simulink model "rx2"  (R2022b)
settings: Solver=FixedStepDiscrete  StartTime=0.0  StopTime=3.3E6  FixedStep=1  RelTol=1e-3  EnableMultiTasking=on
model workspace (MAT data in the model file):
  mwTaskManagerKernelLatency = 0
undefined symbols (not defined in the file or in its folder): Add, jsin, magnitude, rom_pilot_conj_tt, Shift
libraries: hdlsllib x3231, whdlutilities x525, simulink x260, whdlmod x112, whdledac x26, dsphdlmathfun2 x24, commchan3 x1
(part 16 of 59)

== system rx2/process9/decoder/p-p ==
  data_in : Inport  OutDataTypeStr=boolean  PortDimensions=64
  start_in : Inport  Port=2  OutDataTypeStr=boolean  PortDimensions=1
  valid : Inport  Port=3  OutDataTypeStr=boolean  PortDimensions=1
  Compare To Constant : hdlsllib/Logic and Bit Operations/Compare To Constant  relop===  const=64  OutDataTypeStr=boolean
  Compare To Constant1 : hdlsllib/Logic and Bit Operations/Compare To Constant  relop=<=  const=72  OutDataTypeStr=boolean
  Compare To Constant2 : hdlsllib/Logic and Bit Operations/Compare To Constant  relop===  const=1  OutDataTypeStr=boolean
  Compare To Constant3 : hdlsllib/Logic and Bit Operations/Compare To Constant  relop===  const=528  OutDataTypeStr=boolean
  Compare To Constant4 : hdlsllib/Logic and Bit Operations/Compare To Constant  relop=<=  const=528  OutDataTypeStr=boolean
  Delay : Delay  DelayLength=1  InitialCondition=0
  Delay1 : Delay  DelayLength=1  InitialCondition=0
  Ground : Ground
  HDL Counter : hdlsllib/Sources/HDL Counter  CountType=Count limited  CountInit=0  CountStep=1  CountMax=2000  CountFromType=Specify  CountFrom=0  CountResetPort=on  CountLoadPort=off  CountEnbPort=on  CountDirPort=off  CountHitOutputPort=off  CountDataType=Unsigned  CountWordLen=16  CountFracLen=0  CountSampTime=1
  HDL Counter1 : hdlsllib/Sources/HDL Counter  CountType=Count limited  CountInit=1  CountStep=1  CountMax=64  CountFromType=Specify  CountFrom=1  CountResetPort=on  CountLoadPort=off  CountEnbPort=on  CountDirPort=off  CountHitOutputPort=off  CountDataType=Unsigned  CountWordLen=16  CountFracLen=0  CountSampTime=1
  HDL Counter2 : hdlsllib/Sources/HDL Counter  CountType=Count limited  CountInit=0  CountStep=1  CountMax=100  CountFromType=Specify  CountFrom=0  CountResetPort=on  CountLoadPort=off  CountEnbPort=on  CountDirPort=off  CountHitOutputPort=off  CountDataType=Unsigned  CountWordLen=16  CountFracLen=0  CountSampTime=1
  HDL Counter3 : hdlsllib/Sources/HDL Counter  CountType=Count limited  CountInit=1  CountStep=1  CountMax=64*2  CountFromType=Initial value  CountFrom=1  CountResetPort=on  CountLoadPort=off  CountEnbPort=on  CountDirPort=off  CountHitOutputPort=off  CountDataType=Unsigned  CountWordLen=8  CountFracLen=0  CountSampTime=1
  HDL Counter4 : hdlsllib/Sources/HDL Counter  CountType=Count limited  CountInit=0  CountStep=1  CountMax=1000  CountFromType=Initial value  CountFrom=0  CountResetPort=on  CountLoadPort=off  CountEnbPort=on  CountDirPort=off  CountHitOutputPort=off  CountDataType=Unsigned  CountWordLen=16  CountFracLen=0  CountSampTime=1
  HDL Counter5 : hdlsllib/Sources/HDL Counter  CountType=Count limited  CountInit=1  CountStep=1  CountMax=1000  CountFromType=Initial value  CountFrom=1  CountResetPort=on  CountLoadPort=off  CountEnbPort=on  CountDirPort=off  CountHitOutputPort=off  CountDataType=Unsigned  CountWordLen=16  CountFracLen=0  CountSampTime=1
  Logical Operator1 : Logic  Operator=NOT  AllPortsSameDT=off  OutDataTypeStr=boolean
  Logical Operator2 : Logic  Operator=NOT  AllPortsSameDT=off  OutDataTypeStr=boolean
  Logical Operator3 : Logic  AllPortsSameDT=off  OutDataTypeStr=boolean
  Logical Operator5 : Logic  Operator=NOT  AllPortsSameDT=off  OutDataTypeStr=boolean
  Logical Operator6 : Logic  AllPortsSameDT=off  OutDataTypeStr=boolean
  Sample Control Bus Creator : whdlutilities/Sample Control Bus Creator
  Subsystem : Subsystem  mask{valid_length=20*64}
      mask prompts: valid_length "The length of valid"
      mask DialogControl Control2 Prompt: Latency=2
  Subsystem2 : Subsystem  mask{data_type=boolean, address_len=16}
      mask prompts: data_type "the type of input data"; address_len "the length of address"
      mask DialogControl ParameterGroupVar Prompt: 参数
  Switch : Switch  Criteria=u2 ~= 0  SaturateOnIntegerOverflow=off  InputSameDT=off
  p_s_new : Subsystem
  data : Outport
  ctrl : Outport  Port=2
  wires:
  Ground/1 -> Switch/3
  Switch/1 -> data/1
  Subsystem/3(end_out) -> p_s_new/3(end)
  p_s_new/1(data_out) -> Delay1/1
  Subsystem2/1(rd_dout) -> p_s_new/1(data_in)
  Subsystem/1(valid_out) -> HDL Counter1/2, Logical Operator1/1, HDL Counter3/2, Logical Operator2/1, Logical Operator3/1, p_s_new/2(valid)
  Logical Operator6/1 -> HDL Counter4/2, Delay/1
  Compare To Constant4/1 -> Logical Operator6/1
  HDL Counter5/1 -> Compare To Constant4/1
  Sample Control Bus Creator/1 -> ctrl/1
  Delay1/1 -> Switch/1
  Delay/1 -> Sample Control Bus Creator/3, Switch/2
  Compare To Constant3/1 -> HDL Counter4/1, Sample Control Bus Creator/2
  Compare To Constant2/1 -> Sample Control Bus Creator/1
  HDL Counter1/1 -> Compare To Constant/1
  Compare To Constant1/1 -> Logical Operator3/2
  HDL Counter3/1 -> Compare To Constant1/1
  HDL Counter2/1 -> Subsystem2/4(rd_addr)
  data_in/1 -> Subsystem2/1(data1)
  Logical Operator5/1 -> HDL Counter/1
  Logical Operator2/1 -> HDL Counter3/1, HDL Counter5/1
  Compare To Constant/1 -> HDL Counter2/2
  start_in/1 -> Subsystem/1(start)
  HDL Counter/1 -> Subsystem2/2(wr_addr)
  valid/1 -> Logical Operator5/1, Subsystem2/3(wr_en1), HDL Counter/2
  Logical Operator3/1 -> Logical Operator6/2, HDL Counter5/2
  Logical Operator1/1 -> HDL Counter1/1, HDL Counter2/1
  HDL Counter4/1 -> Compare To Constant2/1, Compare To Constant3/1

== system rx2/process9/decoder/rate recover ==
  demod : Inport
  valid_in : Inport  Port=2
  start_in : Inport  Port=3
  Compare To Constant : hdlsllib/Logic and Bit Operations/Compare To Constant  relop=<=  const=384  OutDataTypeStr=boolean
  Compare To Constant1 : hdlsllib/Logic and Bit Operations/Compare To Constant  relop=>=  const=577  OutDataTypeStr=boolean
  Compare To Constant2 : hdlsllib/Logic and Bit Operations/Compare To Constant  relop=<=  const=1776  OutDataTypeStr=boolean
  Compare To Constant3 : hdlsllib/Logic and Bit Operations/Compare To Constant  relop=>=  const=385  OutDataTypeStr=boolean
  Compare To Constant4 : hdlsllib/Logic and Bit Operations/Compare To Constant  relop=<=  const=576  OutDataTypeStr=boolean
  Compare To Constant5 : hdlsllib/Logic and Bit Operations/Compare To Constant  relop=>=  const=1777  OutDataTypeStr=boolean
  Compare To Constant6 : hdlsllib/Logic and Bit Operations/Compare To Constant  relop=<=  const=3600  OutDataTypeStr=boolean
  Constant : Constant  Value=0
  Constant1 : Constant  Value=0
  Delay{,1..4} (5 alike) : Delay  InitialCondition=0
  HDL Counter : hdlsllib/Sources/HDL Counter  CountType=Count limited  CountInit=1  CountStep=1  CountMax=10000  CountFromType=Initial value  CountFrom=1  CountResetPort=on  CountLoadPort=off  CountEnbPort=on  CountDirPort=off  CountHitOutputPort=off  CountDataType=Unsigned  CountWordLen=16  CountFracLen=0  CountSampTime=1
  HDL Counter1 : hdlsllib/Sources/HDL Counter  CountType=Count limited  CountInit=0  CountStep=1  CountMax=10000  CountFromType=Initial value  CountFrom=0  CountResetPort=on  CountLoadPort=off  CountEnbPort=on  CountDirPort=off  CountHitOutputPort=off  CountDataType=Unsigned  CountWordLen=16  CountFracLen=0  CountSampTime=1
  HDL Counter3 : hdlsllib/Sources/HDL Counter  CountType=Count limited  CountInit=1  CountStep=1  CountMax=10000  CountFromType=Initial value  CountFrom=1  CountResetPort=on  CountLoadPort=off  CountEnbPort=on  CountDirPort=off  CountHitOutputPort=off  CountDataType=Unsigned  CountWordLen=16  CountFracLen=0  CountSampTime=1
  Logical Operator : Logic  Operator=NOT  AllPortsSameDT=off  OutDataTypeStr=boolean
  Logical Operator{1,3..4,6..7} (5 alike) : Logic  AllPortsSameDT=off  OutDataTypeStr=boolean
  Logical Operator5 : Logic  Operator=OR  AllPortsSameDT=off  OutDataTypeStr=boolean
  Logical Operator8 : Logic  Operator=NOT  AllPortsSameDT=off  OutDataTypeStr=boolean
  Simple Dual Port RAM : hdlsllib/HDL RAMs/Simple Dual Port RAM  ram_size=16
  Subsystem : Subsystem  mask{valid_length=3600}
      mask prompts: valid_length "The length of valid"
      mask DialogControl Control2 Prompt: Latency=2
  Switch : Switch  Criteria=u2 ~= 0  SaturateOnIntegerOverflow=off  InputSameDT=off
  Switch1 : Switch  Criteria=u2 ~= 0  OutDataTypeStr=fixdt(1,16,9)  SaturateOnIntegerOverflow=off  InputSameDT=off
  rate_recover : Outport  PortDimensions=1
  start_out : Outport  Port=2  OutDataTypeStr=boolean
  end_out : Outport  Port=3  OutDataTypeStr=boolean
  valid_out : Outport  Port=4  OutDataTypeStr=boolean
  wires:
  Compare To Constant5/1 -> Logical Operator4/1
  Logical Operator3/1 -> Delay3/1
  Subsystem/1(valid_out) -> Logical Operator8/1, Logical Operator6/2, Delay/1, HDL Counter3/2
  Constant1/1 -> Switch1/1
  Subsystem/2(start_out) -> Delay1/1  "start"
  Logical Operator/1 -> HDL Counter/1
  Logical Operator1/1 -> Logical Operator5/2
  Compare To Constant3/1 -> Logical Operator3/1
  Subsystem/3(end_out) -> Delay2/1  "end"
  HDL Counter/1 -> Simple Dual Port RAM/2  "wr_addr"
  Compare To Constant6/1 -> Logical Operator4/2
  Compare To Constant1/1 -> Logical Operator1/1
  Compare To Constant2/1 -> Logical Operator1/2
  valid_in/1 -> Simple Dual Port RAM/3, HDL Counter/2, Logical Operator/1
  Delay1/1 -> start_out/1  "start_out"
  Logical Operator7/1 -> Delay4/1  "3"
  Simple Dual Port RAM/1 -> Switch/3  "rd_dout"
  start_in/1 -> Subsystem/1(start)
  Compare To Constant4/1 -> Logical Operator3/2
  Logical Operator4/1 -> Logical Operator7/1
  Constant/1 -> Switch/1
  Switch/1 -> Switch1/3  "2_out"
  Switch1/1 -> rate_recover/1  "data_out"
  Logical Operator5/1 -> Logical Operator6/1
  Compare To Constant/1 -> Logical Operator5/1
  Delay2/1 -> end_out/1  "end_out"
  demod/1 -> Simple Dual Port RAM/1
  Delay/1 -> Logical Operator7/2, valid_out/1  "valid_out"
  Logical Operator8/1 -> HDL Counter1/1, HDL Counter3/1
  HDL Counter3/1 -> Compare To Constant1/1, Compare To Constant/1, Compare To Constant6/1, Compare To Constant5/1, Compare To Constant4/1, Compare To Constant3/1, Compare To Constant2/1  "count"
  Delay3/1 -> Switch/2  "2"
  Delay4/1 -> Switch1/2  "3"
  Logical Operator6/1 -> HDL Counter1/2  "1"
  HDL Counter1/1 -> Simple Dual Port RAM/4  "rd_addr"

== system rx2/process9/decoder/s-p ==
  data_in : Inport
  valid_in : Inport  Port=2
  Compare To Constant1 : hdlsllib/Logic and Bit Operations/Compare To Constant  relop=<=  const=64  OutDataTypeStr=boolean
  Compare To Constant2 : hdlsllib/Logic and Bit Operations/Compare To Constant  relop===  const=2  OutDataTypeStr=boolean
  Compare To Constant3 : hdlsllib/Logic and Bit Operations/Compare To Constant  relop===  const=3  OutDataTypeStr=boolean
  Compare To Constant4 : hdlsllib/Logic and Bit Operations/Compare To Constant  relop===  const=1  OutDataTypeStr=boolean
  Compare To Constant5 : hdlsllib/Logic and Bit Operations/Compare To Constant  relop===  const=100  OutDataTypeStr=boolean
  Constant2 : Constant  Value=2  OutDataTypeStr=uint8
  Constant3 : Constant  Value=zeros(1,56)  OutDataTypeStr=fixdt(1,16,9)
  Delay1 : Delay  DelayLength=1  InitialCondition=0
  Delay4 : Delay  DelayLength=1  InitialCondition=0
  HDL Counter : hdlsllib/Sources/HDL Counter  CountType=Count limited  CountInit=1  CountStep=1  CountMax=72  CountFromType=Initial value  CountFrom=1  CountResetPort=on  CountLoadPort=off  CountEnbPort=on  CountDirPort=off  CountHitOutputPort=off  CountDataType=Unsigned  CountWordLen=8  CountFracLen=0  CountSampTime=1
  HDL Counter1 : hdlsllib/Sources/HDL Counter  CountType=Count limited  CountInit=1  CountStep=1  CountMax=72  CountFromType=Initial value  CountFrom=1  CountResetPort=on  CountLoadPort=off  CountEnbPort=on  CountDirPort=off  CountHitOutputPort=off  CountDataType=Unsigned  CountWordLen=8  CountFracLen=0  CountSampTime=1
  HDL Counter2 : hdlsllib/Sources/HDL Counter  CountType=Count limited  CountInit=1  CountStep=1  CountMax=72  CountFromType=Initial value  CountFrom=1  CountResetPort=on  CountLoadPort=off  CountEnbPort=on  CountDirPort=off  CountHitOutputPort=off  CountDataType=Unsigned  CountWordLen=8  CountFracLen=0  CountSampTime=1
  HDL Counter3 : hdlsllib/Sources/HDL Counter  CountType=Count limited  CountInit=0  CountStep=1  CountMax=200  CountFromType=Initial value  CountFrom=0  CountResetPort=on  CountLoadPort=off  CountEnbPort=on  CountDirPort=off  CountHitOutputPort=off  CountDataType=Unsigned  CountWordLen=8  CountFracLen=0  CountSampTime=1
  Logical Operator{1,5..6,8} (4 alike) : Logic  Operator=NOT  AllPortsSameDT=off  OutDataTypeStr=boolean
  Logical Operator2 : Logic  Operator=XOR  AllPortsSameDT=off  OutDataTypeStr=boolean
  Logical Operator3 : Logic  AllPortsSameDT=off  OutDataTypeStr=boolean
  Logical Operator4 : Logic  AllPortsSameDT=off  OutDataTypeStr=boolean
  Mod : Math  Operator=mod
  Mux : Mux  Inputs=2
  S-P : Subsystem  mask{data_len=64}
      mask prompts: data_len "the length of parallel"
      mask DialogControl ParameterGroupVar Prompt: 参数
  S-P2 : Subsystem  mask{data_len=8}
      mask prompts: data_len "the length of parallel"
      mask DialogControl ParameterGroupVar Prompt: 参数
  Sample Control Bus Creator : whdlutilities/Sample Control Bus Creator
  Switch1 : Switch  Criteria=u2 ~= 0  OutDataTypeStr=Inherit: Inherit via back propagation  SaturateOnIntegerOverflow=off  InputSameDT=off
  data_out : Outport
  ctrl_out : Outport  Port=2
  wires:
  Compare To Constant1/1 -> Logical Operator8/1, Logical Operator3/2
  Logical Operator2/1 -> Delay1/1, HDL Counter3/2  "valid"
  Logical Operator4/1 -> Sample Control Bus Creator/1  "start"
  HDL Counter/1 -> Compare To Constant1/1
  Compare To Constant2/1 -> Logical Operator2/1, Delay4/1
  S-P2/2(valid_out) -> HDL Counter2/2, Logical Operator6/1
  HDL Counter1/1 -> Compare To Constant2/1
  data_in/1 -> S-P2/1(data_in), S-P/1(data_in)
  valid_in/1 -> Logical Operator1/1, Logical Operator3/1, HDL Counter/2
  Sample Control Bus Creator/1 -> ctrl_out/1
  Constant3/1 -> Mux/2
  HDL Counter3/1 -> Mod/1, Compare To Constant4/1, Compare To Constant5/1
  Compare To Constant3/1 -> Logical Operator2/2
  Mod/1 -> Switch1/2
  Switch1/1 -> data_out/1
  Constant2/1 -> Mod/2
  S-P2/1(data_out) -> Mux/1
  Mux/1 -> Switch1/3
  HDL Counter2/1 -> Compare To Constant3/1
  Logical Operator8/1 -> S-P2/2(valid_in)
  S-P/2(valid_out) -> HDL Counter1/2, Logical Operator5/1  "validout"
  S-P/1(data_out) -> Switch1/1
  Logical Operator3/1 -> S-P/2(valid_in)
  Logical Operator1/1 -> HDL Counter/1
  Logical Operator5/1 -> HDL Counter1/1
  Logical Operator6/1 -> HDL Counter2/1
  Compare To Constant5/1 -> Sample Control Bus Creator/2, HDL Counter3/1  "start"
  Compare To Constant4/1 -> Logical Operator4/2
  Delay4/1 -> Logical Operator4/1
  Delay1/1 -> Sample Control Bus Creator/3

== system rx2/process9/decoder/soft demodule ==
  nVar_tt : Inport  OutDataTypeStr=fixdt(0,16,12)
  G_k_1 : Inport  Port=2
  r_k : Inport  Port=3
  start : Inport  Port=4
  valid : Inport  Port=5
  Complex to Real-Imag : ComplexToRealImag
  Constant1 : Constant  Value=2  OutDataTypeStr=uint16
  Constant2 : Constant  Value=2  OutDataTypeStr=uint16
  Constant3 : Constant  Value=0  OutDataTypeStr=uint16
  Constant4 : Constant  Value=0  OutDataTypeStr=uint16
  Data Type Conversion2 : DataTypeConversion  OutDataTypeStr=boolean  SaturateOnIntegerOverflow=off  RndMeth=Floor
  Delay1 : Delay  InitialCondition=0
  Delay2 : Delay  DelayLength=1  InitialCondition=0
  Delay3 : Delay  InitialCondition=0
  Delay4 : Delay  InitialCondition=0
  HDL Counter : hdlsllib/Sources/HDL Counter  CountType=Count limited  CountInit=1  CountStep=1  CountMax=2000  CountFromType=Initial value  CountFrom=1  CountResetPort=on  CountLoadPort=off  CountEnbPort=on  CountDirPort=off  CountHitOutputPort=off  CountDataType=Unsigned  CountWordLen=16  CountFracLen=0  CountSampTime=1
  HDL Counter2 : hdlsllib/Sources/HDL Counter  CountType=Count limited  CountInit=1  CountStep=1  CountMax=2000  CountFromType=Initial value  CountFrom=1  CountResetPort=on  CountLoadPort=off  CountEnbPort=on  CountDirPort=off  CountHitOutputPort=off  CountDataType=Unsigned  CountWordLen=16  CountFracLen=0  CountSampTime=1
  HDL Counter3 : hdlsllib/Sources/HDL Counter  CountType=Count limited  CountInit=0  CountStep=1  CountMax=2000  CountFromType=Initial value  CountFrom=0  CountResetPort=on  CountLoadPort=off  CountEnbPort=on  CountDirPort=off  CountHitOutputPort=off  CountDataType=Unsigned  CountWordLen=16  CountFracLen=0  CountSampTime=1
  HDL Counter5 : hdlsllib/Sources/HDL Counter  CountType=Count limited  CountInit=0  CountStep=1  CountMax=2000  CountFromType=Initial value  CountFrom=0  CountResetPort=on  CountLoadPort=off  CountEnbPort=on  CountDirPort=off  CountHitOutputPort=off  CountDataType=Unsigned  CountWordLen=16  CountFracLen=0  CountSampTime=1
  Logical Operator2 : Logic  AllPortsSameDT=off  OutDataTypeStr=boolean
  Logical Operator3 : Logic  Operator=NOT  AllPortsSameDT=off  OutDataTypeStr=boolean
  Logical Operator4 : Logic  Operator=NOT  AllPortsSameDT=off  OutDataTypeStr=boolean
  Logical Operator5 : Logic  Operator=NOT  AllPortsSameDT=off  OutDataTypeStr=boolean
  Logical Operator6 : Logic  Operator=XOR  AllPortsSameDT=off  OutDataTypeStr=boolean
  Math Reciprocal2 : Math  Operator=reciprocal  SignedPower=on  OutDataTypeStr=fixdt(1,16,12)
  Mod : Math  Operator=mod  SignedPower=on
  Product : Product
  Product1 : Product
  Product10 : Product  OutDataTypeStr=fixdt(1,35,24)
  Product2 : Product  OutDataTypeStr=fixdt(1,35,24)
  Simple Dual Port RAM : hdlsllib/HDL RAMs/Simple Dual Port RAM  ram_size=16
  Simple Dual Port RAM1 : hdlsllib/HDL RAMs/Simple Dual Port RAM  ram_size=16
  Subsystem : Subsystem  mask{valid_length=demod_length}
      mask prompts: valid_length "The length of valid"
      mask DialogControl Control2 Prompt: Latency=2
  Switch : Switch  Criteria=u2 ~= 0  SaturateOnIntegerOverflow=off  InputSameDT=off
  Switch1 : Switch  Criteria=u2 ~= 0  SaturateOnIntegerOverflow=off  InputSameDT=off
  Switch2 : Switch  Criteria=u2 ~= 0  SaturateOnIntegerOverflow=off  InputSameDT=off
  demod : Outport  OutDataTypeStr=fixdt(1,16,9)  VectorParamsAs1DForOutWhenUnconnected=off
  valid_out : Outport  Port=2  OutDataTypeStr=boolean  VectorParamsAs1DForOutWhenUnconnected=off
  start_out : Outport  Port=3  OutDataTypeStr=boolean  VectorParamsAs1DForOutWhenUnconnected=off
  end_out : Outport  Port=4  OutDataTypeStr=boolean  VectorParamsAs1DForOutWhenUnconnected=off
  wires:
  valid/1 -> Switch2/2, Switch1/2, Simple Dual Port RAM1/3, Simple Dual Port RAM/3, HDL Counter2/2, Logical Operator4/1  "valid_tt"
  start/1 -> Subsystem/1(start)
  Logical Operator2/1 -> Logical Operator6/2, HDL Counter3/2  "mod_1"
  Complex to Real-Imag/2 -> Product1/2  "r_k_imag"
  Subsystem/1(valid_out) -> Delay1/1, HDL Counter/2, Logical Operator3/1, Logical Operator2/2, Logical Operator6/1, Logical Operator5/1
  Product/1 -> Switch1/1  "demod_1"
  Product1/1 -> Switch2/1  "demod_0"
  Switch/1 -> demod/1  "demod"
  Mod/1 -> Data Type Conversion2/1  "mod"
  Logical Operator6/1 -> Delay2/1, HDL Counter5/2  "mod_0"
  Complex to Real-Imag/1 -> Product/2  "r_k_real"
  Logical Operator4/1 -> HDL Counter2/1
  HDL Counter3/1 -> Simple Dual Port RAM/4  "rd_addr1"
  Logical Operator5/1 -> HDL Counter5/1, HDL Counter3/1  "rst"
  Logical Operator3/1 -> HDL Counter/1
  Constant1/1 -> Mod/2
  HDL Counter5/1 -> Simple Dual Port RAM1/4  "rd_addr0"
  Simple Dual Port RAM/1 -> Switch/1  "demod_11"
  HDL Counter2/1 -> Simple Dual Port RAM1/2, Simple Dual Port RAM/2  "wr_addr"
  Simple Dual Port RAM1/1 -> Switch/3  "demod_00"
  Data Type Conversion2/1 -> Logical Operator2/1
  Delay1/1 -> valid_out/1  "valid_out"
  HDL Counter/1 -> Mod/1  "count"
  nVar_tt/1 -> Math Reciprocal2/1  "nvar"
  G_k_1/1 -> Product10/2  "G_k_1"
  r_k/1 -> Complex to Real-Imag/1  "r_k"
  Subsystem/2(start_out) -> Delay3/1
  Subsystem/3(end_out) -> Delay4/1
  Delay2/1 -> Switch/2
  Delay3/1 -> start_out/1  "start_out"
  Delay4/1 -> end_out/1  "end_out"
  Math Reciprocal2/1 -> Product10/1  "nvar"
  Product10/1 -> Product2/2
  Product2/1 -> Product1/1, Product/1
  Constant2/1 -> Product2/1
  Constant3/1 -> Switch1/3
  Switch1/1 -> Simple Dual Port RAM/1  "demod1"
  Constant4/1 -> Switch2/3
  Switch2/1 -> Simple Dual Port RAM1/1  "demod0"

== system rx2/process9/decoder/synchronization ==
  chan_est_tt : Inport
  rxSig_tt : Inport  Port=2
  port1_ctrl : Inport  Port=3  OutDataTypeStr=Bus: BUSOFDM1
  port2_ctrl : Inport  Port=4  OutDataTypeStr=Bus: BUSOFDM1
  Bus Selector1 : BusSelector  OutputSignals=signal1,signal2,signal3,signal4,signal5,signal6,signal7,signal8
  Bus Selector2 : BusSelector  OutputSignals=OFDM_ctrl_bf1_process1,OFDM_ctrl_bf1_process2,OFDM_ctrl_bf1_process3,OFDM_ctrl_bf1_process4,OFDM_ctrl_bf1_process5,OFDM_ctrl_bf1_process6,OFDM_ctrl_bf1_process7,OFDM_ctrl_bf1_process8
  Demux : Demux  Outputs=8
  Demux1 : Demux  Outputs=8
  Mux : Mux  Inputs=8
  Mux1 : Mux  Inputs=8
  data_synchronization1 : Subsystem
  data_synchronization2 : Subsystem
  data_synchronization3 : Subsystem
  data_synchronization4 : Subsystem
  data_synchronization5 : Subsystem
  data_synchronization6 : Subsystem
  data_synchronization7 : Subsystem
  data_synchronization8 : Subsystem
  port1_syn : Outport
  port2_syn : Outport  Port=2
  valid_syn : Outport  Port=3
  wires:
  Bus Selector2/3 -> data_synchronization8/4(port2_ctrl)  "<OFDM_ctrl_bf1_process3>"
  Bus Selector2/4 -> data_synchronization7/4(port2_ctrl)  "<OFDM_ctrl_bf1_process4>"
  Bus Selector2/5 -> data_synchronization6/4(port2_ctrl)  "<OFDM_ctrl_bf1_process5>"
  Bus Selector2/6 -> data_synchronization5/4(port2_ctrl)  "<OFDM_ctrl_bf1_process6>"
  Bus Selector2/7 -> data_synchronization4/4(port2_ctrl)  "<OFDM_ctrl_bf1_process7>"
  Bus Selector2/8 -> data_synchronization3/4(port2_ctrl)  "<OFDM_ctrl_bf1_process8>"
  Bus Selector2/2 -> data_synchronization2/4(port2_ctrl)  "<OFDM_ctrl_bf1_process2>"
  Bus Selector2/1 -> data_synchronization1/4(port2_ctrl)  "<OFDM_ctrl_bf1_process1>"
  port2_ctrl/1 -> Bus Selector2/1
  Bus Selector1/8 -> data_synchronization8/3(port1_ctrl)  "<signal8>"
  Bus Selector1/7 -> data_synchronization7/3(port1_ctrl)  "<signal7>"
  Bus Selector1/6 -> data_synchronization6/3(port1_ctrl)  "<signal6>"
  Bus Selector1/5 -> data_synchronization5/3(port1_ctrl)  "<signal5>"
  Bus Selector1/4 -> data_synchronization4/3(port1_ctrl)  "<signal4>"
  Bus Selector1/3 -> data_synchronization3/3(port1_ctrl)  "<signal3>"
  Bus Selector1/2 -> data_synchronization2/3(port1_ctrl)  "<signal2>"
  Bus Selector1/1 -> data_synchronization1/3(port1_ctrl)  "<signal1>"
  port1_ctrl/1 -> Bus Selector1/1
  rxSig_tt/1 -> Demux1/1
  data_synchronization6/3(valid_syn) -> ?
  chan_est_tt/1 -> Demux/1
  data_synchronization4/4(start_syn) -> ?
  data_synchronization2/3(valid_syn) -> ?
  data_synchronization4/3(valid_syn) -> ?
  data_synchronization6/4(start_syn) -> ?
  data_synchronization7/3(valid_syn) -> ?
  data_synchronization3/3(valid_syn) -> ?
  data_synchronization5/3(valid_syn) -> ?
  data_synchronization8/4(start_syn) -> ?
  Demux1/5 -> data_synchronization5/2(port2)
  Demux1/3 -> data_synchronization3/2(port2)
  data_synchronization2/4(start_syn) -> ?
  data_synchronization3/2(port2_syn) -> Mux1/3
  data_synchronization7/1(port1_syn) -> Mux/7
  Demux1/1 -> data_synchronization1/2(port2)
  Demux/8 -> data_synchronization8/1(port1)
  data_synchronization1/1(port1_syn) -> Mux/1
  Demux/3 -> data_synchronization3/1(port1)
  data_synchronization3/4(start_syn) -> ?
  data_synchronization1/3(valid_syn) -> valid_syn/1
  data_synchronization1/2(port2_syn) -> Mux1/1
  Demux/4 -> data_synchronization4/1(port1)
  data_synchronization5/4(start_syn) -> ?
  data_synchronization8/1(port1_syn) -> Mux/8
  Demux/6 -> data_synchronization6/1(port1)
  data_synchronization7/2(port2_syn) -> Mux1/7
  data_synchronization6/1(port1_syn) -> Mux/6
  Demux/7 -> data_synchronization7/1(port1)
  Demux/1 -> data_synchronization1/1(port1)
  data_synchronization4/2(port2_syn) -> Mux1/4
  data_synchronization4/1(port1_syn) -> Mux/4
  data_synchronization5/2(port2_syn) -> Mux1/5
  data_synchronization5/1(port1_syn) -> Mux/5
  Mux1/1 -> port2_syn/1
  Demux1/4 -> data_synchronization4/2(port2)
  Demux1/6 -> data_synchronization6/2(port2)
  data_synchronization8/2(port2_syn) -> Mux1/8
  data_synchronization2/2(port2_syn) -> Mux1/2
  data_synchronization7/4(start_syn) -> ?
  data_synchronization6/2(port2_syn) -> Mux1/6
  Demux/5 -> data_synchronization5/1(port1)
  Demux1/8 -> data_synchronization8/2(port2)
  data_synchronization8/3(valid_syn) -> ?
  Demux1/7 -> data_synchronization7/2(port2)
  data_synchronization2/1(port1_syn) -> Mux/2
  Mux/1 -> port1_syn/1
  Demux1/2 -> data_synchronization2/2(port2)
  Demux/2 -> data_synchronization2/1(port1)
  data_synchronization3/1(port1_syn) -> Mux/3

== system rx2/process9/decoder/synchronize_valid ==
  start : Inport
  Compare To Constant : simulink/Logic and Bit Operations/Compare To Constant  relop===  const=valid_length  OutDataTypeStr=boolean
  Data Type Conversion : DataTypeConversion  OutDataTypeStr=boolean  SaturateOnIntegerOverflow=off  RndMeth=Floor
  Delay2 : Delay  DelayLength=1  InitialCondition=0
  HDL Counter1 : hdlsllib/Sources/HDL Counter  CountType=Count limited  CountInit=1  CountStep=1  CountMax=valid_length  CountFromType=Initial value  CountFrom=1  CountResetPort=off  CountLoadPort=off  CountEnbPort=on  CountDirPort=off  CountHitOutputPort=off  CountDataType=Unsigned  CountWordLen=16  CountFracLen=0  CountSampTime=1
  HDL Counter4 : hdlsllib/Sources/HDL Counter  CountType=Count limited  CountInit=0  CountStep=1  CountMax=1  CountFromType=Initial value  CountFrom=0  CountResetPort=on  CountLoadPort=off  CountEnbPort=on  CountDirPort=off  CountHitOutputPort=off  CountDataType=Unsigned  CountWordLen=8  CountFracLen=0  CountSampTime=1
  valid_out : Outport
  wires:
  Compare To Constant/1 -> HDL Counter4/1
  HDL Counter1/1 -> Compare To Constant/1  "count_1"
  HDL Counter4/1 -> Data Type Conversion/1
  start/1 -> HDL Counter4/2
  Data Type Conversion/1 -> Delay2/1, HDL Counter1/1
  Delay2/1 -> valid_out/1  "valid_out"

== system rx2/demode1/chan_est1/Subsystem/HDL_DUT ==
  data_in : Inport  OutDataTypeStr=fixdt(1,16,12)
  ctrl_in : Inport  Port=2  OutDataTypeStr=Bus: samplecontrol
  Bus Selector : BusSelector  OutputSignals=start,end,valid
  Delay : Delay  InitialCondition=0
  Delay1 : Delay  InitialCondition=0
  Ground : Ground
  H_est : Subsystem
  LS_Est : Subsystem
  Pliot : Subsystem
  Switch : Switch  Criteria=u2 ~= 0  SaturateOnIntegerOverflow=off  InputSameDT=off
  TA_EST : Subsystem
  delta_estimator : Subsystem
  H_out : Outport  OutDataTypeStr=fixdt(1,32,27)  VectorParamsAs1DForOutWhenUnconnected=off
  w_out : Outport  Port=2  VectorParamsAs1DForOutWhenUnconnected=off
  ctrl_out : Outport  Port=3  OutDataTypeStr=Bus:samplecontrol  VectorParamsAs1DForOutWhenUnconnected=off
  wires:
  data_in/1 -> Delay/1
  H_est/1(H_out) -> H_out/1
  Pliot/1(pilot) -> LS_Est/2(LS_polit_in)
  ctrl_in/1 -> Bus Selector/1
  Bus Selector/3 -> Pliot/1(enb), Delay1/1  "<valid>"
  H_est/2(H_valid_out) -> ctrl_out/1
  LS_Est/1(LS_result_out) -> TA_EST/1(data_in)  "result"
  LS_Est/2(LS_ctrl_out) -> TA_EST/2(ctrl_in)  "valid1"
  TA_EST/1(hta_est_data) -> H_est/1(H_result_in)
  TA_EST/2(hta_est_ctrl) -> H_est/2(H_ctrl_in)
  Delay/1 -> LS_Est/1(LS_data_in)
  Delay1/1 -> LS_Est/3(LS_valid_in)
  delta_estimator/1(data_out) -> w_out/1
  LS_Est/3(wdata_out) -> Switch/1
  LS_Est/4(wvalid_out) -> delta_estimator/2(valid_in), Switch/2
  Ground/1 -> Switch/3
  Switch/1 -> delta_estimator/1(data_in)

== system rx2/demode1/chan_est1/Subsystem/HDL_DUT1 ==
  data_in : Inport  OutDataTypeStr=fixdt(1,16,12)
  ctrl_in : Inport  Port=2  OutDataTypeStr=Bus: samplecontrol
  Bus Selector : BusSelector  OutputSignals=start,end,valid
  Delay : Delay  InitialCondition=0
  Delay1 : Delay  InitialCondition=0
  Ground : Ground
  H_est : Subsystem
  LS_Est : Subsystem
  Pliot : Subsystem
  Switch : Switch  Criteria=u2 ~= 0  SaturateOnIntegerOverflow=off  InputSameDT=off
  TA_EST : Subsystem
  delta_estimator : Subsystem
  H_out : Outport  OutDataTypeStr=fixdt(1,32,27)  VectorParamsAs1DForOutWhenUnconnected=off
  w_out : Outport  Port=2  VectorParamsAs1DForOutWhenUnconnected=off
  ctrl_out : Outport  Port=3  OutDataTypeStr=Bus:samplecontrol  VectorParamsAs1DForOutWhenUnconnected=off
  wires:
  data_in/1 -> Delay/1
  H_est/1(H_out) -> H_out/1
  Pliot/1(pilot) -> LS_Est/2(LS_polit_in)
  ctrl_in/1 -> Bus Selector/1
  Bus Selector/3 -> Pliot/1(enb), Delay1/1  "<valid>"
  H_est/2(H_valid_out) -> ctrl_out/1
  LS_Est/1(LS_result_out) -> TA_EST/1(data_in)  "result"
  LS_Est/2(LS_ctrl_out) -> TA_EST/2(ctrl_in)  "valid1"
  TA_EST/1(hta_est_data) -> H_est/1(H_result_in)
  TA_EST/2(hta_est_ctrl) -> H_est/2(H_ctrl_in)
  Delay/1 -> LS_Est/1(LS_data_in)
  Delay1/1 -> LS_Est/3(LS_valid_in)
  delta_estimator/1(data_out) -> w_out/1
  LS_Est/3(wdata_out) -> Switch/1
  LS_Est/4(wvalid_out) -> delta_estimator/2(valid_in), Switch/2
  Ground/1 -> Switch/3
  Switch/1 -> delta_estimator/1(data_in)

== system rx2/demode1/chan_est1/Subsystem/HDL_DUT2 ==
  data_in : Inport  OutDataTypeStr=fixdt(1,16,12)
  ctrl_in : Inport  Port=2  OutDataTypeStr=Bus: samplecontrol
  Bus Selector : BusSelector  OutputSignals=start,end,valid
  Delay : Delay  InitialCondition=0
  Delay1 : Delay  InitialCondition=0
  Ground : Ground
  H_est : Subsystem
  LS_Est : Subsystem
  Pliot : Subsystem
  Switch : Switch  Criteria=u2 ~= 0  SaturateOnIntegerOverflow=off  InputSameDT=off
  TA_EST : Subsystem
  delta_estimator : Subsystem
  H_out : Outport  OutDataTypeStr=fixdt(1,32,27)  VectorParamsAs1DForOutWhenUnconnected=off
  w_out : Outport  Port=2  VectorParamsAs1DForOutWhenUnconnected=off
  ctrl_out : Outport  Port=3  OutDataTypeStr=Bus:samplecontrol  VectorParamsAs1DForOutWhenUnconnected=off
  wires:
  data_in/1 -> Delay/1
  H_est/1(H_out) -> H_out/1
  Pliot/1(pilot) -> LS_Est/2(LS_polit_in)
  ctrl_in/1 -> Bus Selector/1
  Bus Selector/3 -> Pliot/1(enb), Delay1/1  "<valid>"
  H_est/2(H_valid_out) -> ctrl_out/1
  LS_Est/1(LS_result_out) -> TA_EST/1(data_in)  "result"
  LS_Est/2(LS_ctrl_out) -> TA_EST/2(ctrl_in)  "valid1"
  TA_EST/1(hta_est_data) -> H_est/1(H_result_in)
  TA_EST/2(hta_est_ctrl) -> H_est/2(H_ctrl_in)
  Delay/1 -> LS_Est/1(LS_data_in)
  Delay1/1 -> LS_Est/3(LS_valid_in)
  delta_estimator/1(data_out) -> w_out/1
  LS_Est/3(wdata_out) -> Switch/1
  LS_Est/4(wvalid_out) -> delta_estimator/2(valid_in), Switch/2
  Ground/1 -> Switch/3
  Switch/1 -> delta_estimator/1(data_in)

== system rx2/demode1/chan_est1/Subsystem/HDL_DUT3 ==
  data_in : Inport  OutDataTypeStr=fixdt(1,16,12)
  ctrl_in : Inport  Port=2  OutDataTypeStr=Bus: samplecontrol
  Bus Selector : BusSelector  OutputSignals=start,end,valid
  Delay : Delay  InitialCondition=0
  Delay1 : Delay  InitialCondition=0
  Ground : Ground
  H_est : Subsystem
  LS_Est : Subsystem
  Pliot : Subsystem
  Switch : Switch  Criteria=u2 ~= 0  SaturateOnIntegerOverflow=off  InputSameDT=off
  TA_EST : Subsystem
  delta_estimator : Subsystem
  H_out : Outport  OutDataTypeStr=fixdt(1,32,27)  VectorParamsAs1DForOutWhenUnconnected=off
  w_out : Outport  Port=2  VectorParamsAs1DForOutWhenUnconnected=off
  ctrl_out : Outport  Port=3  OutDataTypeStr=Bus:samplecontrol  VectorParamsAs1DForOutWhenUnconnected=off
  wires:
  data_in/1 -> Delay/1
  H_est/1(H_out) -> H_out/1
  Pliot/1(pilot) -> LS_Est/2(LS_polit_in)
  ctrl_in/1 -> Bus Selector/1
  Bus Selector/3 -> Pliot/1(enb), Delay1/1  "<valid>"
  H_est/2(H_valid_out) -> ctrl_out/1
  LS_Est/1(LS_result_out) -> TA_EST/1(data_in)  "result"
  LS_Est/2(LS_ctrl_out) -> TA_EST/2(ctrl_in)  "valid1"
  TA_EST/1(hta_est_data) -> H_est/1(H_result_in)
  TA_EST/2(hta_est_ctrl) -> H_est/2(H_ctrl_in)
  Delay/1 -> LS_Est/1(LS_data_in)
  Delay1/1 -> LS_Est/3(LS_valid_in)
  delta_estimator/1(data_out) -> w_out/1
  LS_Est/3(wdata_out) -> Switch/1
  LS_Est/4(wvalid_out) -> delta_estimator/2(valid_in), Switch/2
  Ground/1 -> Switch/3
  Switch/1 -> delta_estimator/1(data_in)

== system rx2/demode1/chan_est1/Subsystem/HDL_DUT4 ==
  data_in : Inport  OutDataTypeStr=fixdt(1,16,12)
  ctrl_in : Inport  Port=2  OutDataTypeStr=Bus: samplecontrol
  Bus Selector : BusSelector  OutputSignals=start,end,valid
  Delay : Delay  InitialCondition=0
  Delay1 : Delay  InitialCondition=0
  Ground : Ground
  H_est : Subsystem
  LS_Est : Subsystem
  Pliot : Subsystem
  Switch : Switch  Criteria=u2 ~= 0  SaturateOnIntegerOverflow=off  InputSameDT=off
  TA_EST : Subsystem
  delta_estimator : Subsystem
  H_out : Outport  OutDataTypeStr=fixdt(1,32,27)  VectorParamsAs1DForOutWhenUnconnected=off
  w_out : Outport  Port=2  VectorParamsAs1DForOutWhenUnconnected=off
  ctrl_out : Outport  Port=3  OutDataTypeStr=Bus:samplecontrol  VectorParamsAs1DForOutWhenUnconnected=off
  wires:
  data_in/1 -> Delay/1
  H_est/1(H_out) -> H_out/1
  Pliot/1(pilot) -> LS_Est/2(LS_polit_in)
  ctrl_in/1 -> Bus Selector/1
  Bus Selector/3 -> Pliot/1(enb), Delay1/1  "<valid>"
  H_est/2(H_valid_out) -> ctrl_out/1
  LS_Est/1(LS_result_out) -> TA_EST/1(data_in)  "result"
  LS_Est/2(LS_ctrl_out) -> TA_EST/2(ctrl_in)  "valid1"
  TA_EST/1(hta_est_data) -> H_est/1(H_result_in)
  TA_EST/2(hta_est_ctrl) -> H_est/2(H_ctrl_in)
  Delay/1 -> LS_Est/1(LS_data_in)
  Delay1/1 -> LS_Est/3(LS_valid_in)
  delta_estimator/1(data_out) -> w_out/1
  LS_Est/3(wdata_out) -> Switch/1
  LS_Est/4(wvalid_out) -> delta_estimator/2(valid_in), Switch/2
  Ground/1 -> Switch/3
  Switch/1 -> delta_estimator/1(data_in)

== system rx2/demode1/chan_est1/Subsystem/HDL_DUT5 ==
  data_in : Inport  OutDataTypeStr=fixdt(1,16,12)
  ctrl_in : Inport  Port=2  OutDataTypeStr=Bus: samplecontrol
  Bus Selector : BusSelector  OutputSignals=start,end,valid
  Delay : Delay  InitialCondition=0
  Delay1 : Delay  InitialCondition=0
  Ground : Ground
  H_est : Subsystem
  LS_Est : Subsystem
  Pliot : Subsystem
  Switch : Switch  Criteria=u2 ~= 0  SaturateOnIntegerOverflow=off  InputSameDT=off
  TA_EST : Subsystem
  delta_estimator : Subsystem
  H_out : Outport  OutDataTypeStr=fixdt(1,32,27)  VectorParamsAs1DForOutWhenUnconnected=off
  w_out : Outport  Port=2  VectorParamsAs1DForOutWhenUnconnected=off
  ctrl_out : Outport  Port=3  OutDataTypeStr=Bus:samplecontrol  VectorParamsAs1DForOutWhenUnconnected=off
  wires:
  data_in/1 -> Delay/1
  H_est/1(H_out) -> H_out/1
  Pliot/1(pilot) -> LS_Est/2(LS_polit_in)
  ctrl_in/1 -> Bus Selector/1
  Bus Selector/3 -> Pliot/1(enb), Delay1/1  "<valid>"
  H_est/2(H_valid_out) -> ctrl_out/1
  LS_Est/1(LS_result_out) -> TA_EST/1(data_in)  "result"
  LS_Est/2(LS_ctrl_out) -> TA_EST/2(ctrl_in)  "valid1"
  TA_EST/1(hta_est_data) -> H_est/1(H_result_in)
  TA_EST/2(hta_est_ctrl) -> H_est/2(H_ctrl_in)
  Delay/1 -> LS_Est/1(LS_data_in)
  Delay1/1 -> LS_Est/3(LS_valid_in)
  delta_estimator/1(data_out) -> w_out/1
  LS_Est/3(wdata_out) -> Switch/1
  LS_Est/4(wvalid_out) -> delta_estimator/2(valid_in), Switch/2
  Ground/1 -> Switch/3
  Switch/1 -> delta_estimator/1(data_in)

== system rx2/demode1/chan_est1/Subsystem/HDL_DUT6 ==
  data_in : Inport  OutDataTypeStr=fixdt(1,16,12)
  ctrl_in : Inport  Port=2  OutDataTypeStr=Bus: samplecontrol
  Bus Selector : BusSelector  OutputSignals=start,end,valid
  Delay : Delay  InitialCondition=0
  Delay1 : Delay  InitialCondition=0
  Ground : Ground
  H_est : Subsystem
  LS_Est : Subsystem
  Pliot : Subsystem
  Switch : Switch  Criteria=u2 ~= 0  SaturateOnIntegerOverflow=off  InputSameDT=off
  TA_EST : Subsystem
  delta_estimator : Subsystem
  H_out : Outport  OutDataTypeStr=fixdt(1,32,27)  VectorParamsAs1DForOutWhenUnconnected=off
  w_out : Outport  Port=2  VectorParamsAs1DForOutWhenUnconnected=off
  ctrl_out : Outport  Port=3  OutDataTypeStr=Bus:samplecontrol  VectorParamsAs1DForOutWhenUnconnected=off
  wires:
  data_in/1 -> Delay/1
  H_est/1(H_out) -> H_out/1
  Pliot/1(pilot) -> LS_Est/2(LS_polit_in)
  ctrl_in/1 -> Bus Selector/1
  Bus Selector/3 -> Pliot/1(enb), Delay1/1  "<valid>"
  H_est/2(H_valid_out) -> ctrl_out/1
  LS_Est/1(LS_result_out) -> TA_EST/1(data_in)  "result"
  LS_Est/2(LS_ctrl_out) -> TA_EST/2(ctrl_in)  "valid1"
  TA_EST/1(hta_est_data) -> H_est/1(H_result_in)
  TA_EST/2(hta_est_ctrl) -> H_est/2(H_ctrl_in)
  Delay/1 -> LS_Est/1(LS_data_in)
  Delay1/1 -> LS_Est/3(LS_valid_in)
  delta_estimator/1(data_out) -> w_out/1
  LS_Est/3(wdata_out) -> Switch/1
  LS_Est/4(wvalid_out) -> delta_estimator/2(valid_in), Switch/2
  Ground/1 -> Switch/3
  Switch/1 -> delta_estimator/1(data_in)

== system rx2/demode1/chan_est1/Subsystem/HDL_DUT7 ==
  data_in : Inport  OutDataTypeStr=fixdt(1,16,12)
  ctrl_in : Inport  Port=2  OutDataTypeStr=Bus: samplecontrol
  Bus Selector : BusSelector  OutputSignals=start,end,valid
  Delay : Delay  InitialCondition=0
  Delay1 : Delay  InitialCondition=0
  Ground : Ground
  H_est : Subsystem
  LS_Est : Subsystem
  Pliot : Subsystem
  Switch : Switch  Criteria=u2 ~= 0  SaturateOnIntegerOverflow=off  InputSameDT=off
  TA_EST : Subsystem
  delta_estimator : Subsystem
  H_out : Outport  OutDataTypeStr=fixdt(1,32,27)  VectorParamsAs1DForOutWhenUnconnected=off
  w_out : Outport  Port=2  VectorParamsAs1DForOutWhenUnconnected=off
  ctrl_out : Outport  Port=3  OutDataTypeStr=Bus:samplecontrol  VectorParamsAs1DForOutWhenUnconnected=off
  wires:
  data_in/1 -> Delay/1
  H_est/1(H_out) -> H_out/1
  Pliot/1(pilot) -> LS_Est/2(LS_polit_in)
  ctrl_in/1 -> Bus Selector/1
  Bus Selector/3 -> Pliot/1(enb), Delay1/1  "<valid>"
  H_est/2(H_valid_out) -> ctrl_out/1
  LS_Est/1(LS_result_out) -> TA_EST/1(data_in)  "result"
  LS_Est/2(LS_ctrl_out) -> TA_EST/2(ctrl_in)  "valid1"
  TA_EST/1(hta_est_data) -> H_est/1(H_result_in)
  TA_EST/2(hta_est_ctrl) -> H_est/2(H_ctrl_in)
  Delay/1 -> LS_Est/1(LS_data_in)
  Delay1/1 -> LS_Est/3(LS_valid_in)
  delta_estimator/1(data_out) -> w_out/1
  LS_Est/3(wdata_out) -> Switch/1
  LS_Est/4(wvalid_out) -> delta_estimator/2(valid_in), Switch/2
  Ground/1 -> Switch/3
  Switch/1 -> delta_estimator/1(data_in)

== system rx2/demode1/chan_est1/Subsystem/OFDM_DEMOD1 ==
  process : Inport
  process_ctrl : Inport  Port=2  OutDataTypeStr=Bus: BUSOFDM1
  Bus Selector : BusSelector  OutputSignals=signal1 (signal 1).valid,signal1 (signal 2).valid,signal1 (signal 3).valid,signal1 (signal 4).valid,signal1 (signal 5).valid,signal1 (signal 6).valid,signal1 (signal 7).valid,signal1 (signal 8).valid
  Demux : Demux  Outputs=8
  OFDM_demod1 : Subsystem
  OFDM_demod2 : Subsystem
  OFDM_demod3 : Subsystem
  OFDM_demod4 : Subsystem
  OFDM_demod5 : Subsystem
  OFDM_demod6 : Subsystem
  OFDM_demod7 : Subsystem
  OFDM_demod8 : Subsystem
  data_in : Outport
  OFDM_ctrl_bf1_process1 : Outport  Port=2
  Out3 : Outport  Port=3
  OFDM_ctrl_bf1_process2 : Outport  Port=4
  Out5 : Outport  Port=5
  OFDM_ctrl_bf1_process3 : Outport  Port=6
  Out7 : Outport  Port=7
  OFDM_ctrl_bf1_process4 : Outport  Port=8
  Out9 : Outport  Port=9
  OFDM_ctrl_bf1_process5 : Outport  Port=10
  Out11 : Outport  Port=11
  OFDM_ctrl_bf1_process6 : Outport  Port=12
  Out13 : Outport  Port=13
  OFDM_ctrl_bf1_process7 : Outport  Port=14
  Out15 : Outport  Port=15
  OFDM_ctrl_bf1_process8 : Outport  Port=16
  wires:
  process_ctrl/1 -> Bus Selector/1
  process/1 -> Demux/1
  Demux/1 -> OFDM_demod1/1(ofdm_sym)
  Demux/2 -> OFDM_demod2/1(ofdm_sym)
  Bus Selector/2 -> OFDM_demod2/2(valid_in)  "<valid>"
  Demux/3 -> OFDM_demod3/1(ofdm_sym)
  Bus Selector/3 -> OFDM_demod3/2(valid_in)  "<valid>"
  Demux/4 -> OFDM_demod4/1(ofdm_sym)
  Bus Selector/4 -> OFDM_demod4/2(valid_in)  "<valid>"
  Bus Selector/5 -> OFDM_demod5/2(valid_in)  "<valid>"
  Bus Selector/6 -> OFDM_demod6/2(valid_in)  "<valid>"
  Bus Selector/7 -> OFDM_demod8/2(valid_in)  "<valid>"
  Bus Selector/8 -> OFDM_demod7/2(valid_in)  "<valid>"
  Demux/5 -> OFDM_demod5/1(ofdm_sym)
  Demux/6 -> OFDM_demod6/1(ofdm_sym)
  Demux/7 -> OFDM_demod8/1(ofdm_sym)
  Demux/8 -> OFDM_demod7/1(ofdm_sym)
  Bus Selector/1 -> OFDM_demod1/2(valid_in)  "<valid>"
  OFDM_demod5/2(ctrl_out) -> OFDM_ctrl_bf1_process5/1  "OFDM_ctrl_bf1_process5"
  OFDM_demod2/1(data_out) -> Out3/1
  OFDM_demod7/2(ctrl_out) -> OFDM_ctrl_bf1_process8/1  "OFDM_ctrl_bf1_process8"
  OFDM_demod3/1(data_out) -> Out5/1
  OFDM_demod3/2(ctrl_out) -> OFDM_ctrl_bf1_process3/1  "OFDM_ctrl_bf1_process3"
  OFDM_demod8/2(ctrl_out) -> OFDM_ctrl_bf1_process7/1  "OFDM_ctrl_bf1_process7"
  OFDM_demod5/1(data_out) -> Out9/1
  OFDM_demod1/1(data_out) -> data_in/1
  OFDM_demod2/2(ctrl_out) -> OFDM_ctrl_bf1_process2/1  "OFDM_ctrl_bf1_process2"
  OFDM_demod6/2(ctrl_out) -> OFDM_ctrl_bf1_process6/1  "OFDM_ctrl_bf1_process6"
  OFDM_demod8/1(data_out) -> Out13/1
  OFDM_demod6/1(data_out) -> Out11/1
  OFDM_demod4/2(ctrl_out) -> OFDM_ctrl_bf1_process4/1  "OFDM_ctrl_bf1_process4"
  OFDM_demod1/2(ctrl_out) -> OFDM_ctrl_bf1_process1/1  "OFDM_ctrl_bf1_process1"
  OFDM_demod4/1(data_out) -> Out7/1
  OFDM_demod7/1(data_out) -> Out15/1

== system rx2/demode1/chan_est1/Subsystem/Subsystem1 ==
  H_out : Inport
  w_out : Inport  Port=2
  In3 : Inport  Port=3
  H_out1 : Inport  Port=4
  w_out1 : Inport  Port=5
  ctrl_out : Inport  Port=6
  H_out2 : Inport  Port=7
  w_out2 : Inport  Port=8
  In9 : Inport  Port=9
  H_out3 : Inport  Port=10
  w_out3 : Inport  Port=11
  In12 : Inport  Port=12
  H_out4 : Inport  Port=13
  w_out4 : Inport  Port=14
  In15 : Inport  Port=15
  H_out5 : Inport  Port=16
  w_out5 : Inport  Port=17
  In18 : Inport  Port=18
  H_out6 : Inport  Port=19
  w_out6 : Inport  Port=20
  In21 : Inport  Port=21
  H_out7 : Inport  Port=22
  w_out7 : Inport  Port=23
  In24 : Inport  Port=24
  Bus Creator : BusCreator  Inputs=8
  Constant1 : Constant  Value=1/8  OutDataTypeStr=fixdt(1,40,24)  SampleTime=-1
  Data Type Conversion : DataTypeConversion  OutDataTypeStr=fixdt(1,16,12)  SaturateOnIntegerOverflow=off  RndMeth=Floor
  Divide : Product  Inputs=**  OutDataTypeStr=fixdt(0,16,12)  RndMeth=Zero  SaturateOnIntegerOverflow=on
  Mux : Mux  Inputs=8
  Sum : Sum  Inputs=++++++++
  Out1 : Outport  OutDataTypeStr=fixdt(1,16,12)
  Out3 : Outport  Port=2  OutDataTypeStr=Bus: BUSOFDM1
  σ² : Outport  Port=3  OutDataTypeStr=fixdt(0,16,12)
  wires:
  Sum/1 -> Divide/1
  w_out4/1 -> Sum/5
  In21/1 -> Bus Creator/7
  H_out2/1 -> Mux/3
  Mux/1 -> Data Type Conversion/1
  Constant1/1 -> Divide/2
  H_out7/1 -> Mux/8
  In9/1 -> Bus Creator/3
  w_out/1 -> Sum/1
  In18/1 -> Bus Creator/6
  H_out5/1 -> Mux/6
  H_out3/1 -> Mux/4
  ctrl_out/1 -> Bus Creator/2
  w_out5/1 -> Sum/6
  In24/1 -> Bus Creator/8
  Bus Creator/1 -> Out3/1
  w_out2/1 -> Sum/3
  In3/1 -> Bus Creator/1
  H_out1/1 -> Mux/2
  w_out3/1 -> Sum/4
  w_out1/1 -> Sum/2
  In12/1 -> Bus Creator/4
  w_out6/1 -> Sum/7
  H_out/1 -> Mux/1
  H_out4/1 -> Mux/5
  w_out7/1 -> Sum/8
  H_out6/1 -> Mux/7
  Divide/1 -> σ²/1
  In15/1 -> Bus Creator/5
  Data Type Conversion/1 -> Out1/1

== system rx2/process divide/transport_block1/Subsystem1/ctrl_gen ==
  data_in : Inport
  valid_in : Inport  Port=2
  Delay : Delay  DelayLength=1  InitialCondition=0
  Delay1 : Delay  DelayLength=1  InitialCondition=0
  Delay2 : Delay  DelayLength=1  InitialCondition=0
  Detect Fall Nonpositive : hdlsllib/Logic and Bit Operations/Detect Fall Nonpositive  vinit=0  OutDataTypeStr=boolean
  Detect Rise Positive : hdlsllib/Logic and Bit Operations/Detect Rise Positive  vinit=0  OutDataTypeStr=boolean
  Sample Control Bus Creator : whdlutilities/Sample Control Bus Creator
  data_out : Outport
  ctrl_out : Outport  Port=2
  wires:
  Detect Fall Nonpositive/1 -> Sample Control Bus Creator/2
  valid_in/1 -> Delay/1, Detect Fall Nonpositive/1, Delay1/1
  Sample Control Bus Creator/1 -> ctrl_out/1
  Delay/1 -> Sample Control Bus Creator/3
  Delay1/1 -> Detect Rise Positive/1
  data_in/1 -> Delay2/1
  Delay2/1 -> data_out/1
  Detect Rise Positive/1 -> Sample Control Bus Creator/1

== system rx2/process divide/transport_block1/Subsystem10/ctrl_gen ==
  data_in : Inport
  valid_in : Inport  Port=2
  Delay : Delay  DelayLength=1  InitialCondition=0
  Delay1 : Delay  DelayLength=1  InitialCondition=0
  Delay2 : Delay  DelayLength=1  InitialCondition=0
  Detect Fall Nonpositive : hdlsllib/Logic and Bit Operations/Detect Fall Nonpositive  vinit=0  OutDataTypeStr=boolean
  Detect Rise Positive : hdlsllib/Logic and Bit Operations/Detect Rise Positive  vinit=0  OutDataTypeStr=boolean
  Sample Control Bus Creator : whdlutilities/Sample Control Bus Creator
  data_out : Outport
  ctrl_out : Outport  Port=2
  wires:
  Detect Rise Positive/1 -> Sample Control Bus Creator/1
  Delay2/1 -> data_out/1
  data_in/1 -> Delay2/1
  Delay1/1 -> Detect Rise Positive/1
  Delay/1 -> Sample Control Bus Creator/3
  Sample Control Bus Creator/1 -> ctrl_out/1
  valid_in/1 -> Delay1/1, Detect Fall Nonpositive/1, Delay/1
  Detect Fall Nonpositive/1 -> Sample Control Bus Creator/2

== system rx2/process divide/transport_block1/Subsystem11/ctrl_gen ==
  data_in : Inport
  valid_in : Inport  Port=2
  Delay : Delay  DelayLength=1  InitialCondition=0
  Delay1 : Delay  DelayLength=1  InitialCondition=0
  Delay2 : Delay  DelayLength=1  InitialCondition=0
  Detect Fall Nonpositive : hdlsllib/Logic and Bit Operations/Detect Fall Nonpositive  vinit=0  OutDataTypeStr=boolean
  Detect Rise Positive : hdlsllib/Logic and Bit Operations/Detect Rise Positive  vinit=0  OutDataTypeStr=boolean
  Sample Control Bus Creator : whdlutilities/Sample Control Bus Creator
  data_out : Outport
  ctrl_out : Outport  Port=2
  wires:
  Detect Rise Positive/1 -> Sample Control Bus Creator/1
  Delay2/1 -> data_out/1
  data_in/1 -> Delay2/1
  Delay1/1 -> Detect Rise Positive/1
  Delay/1 -> Sample Control Bus Creator/3
  Sample Control Bus Creator/1 -> ctrl_out/1
  valid_in/1 -> Delay1/1, Detect Fall Nonpositive/1, Delay/1
  Detect Fall Nonpositive/1 -> Sample Control Bus Creator/2

== system rx2/process divide/transport_block1/Subsystem12/ctrl_gen ==
  data_in : Inport
  valid_in : Inport  Port=2
  Delay : Delay  DelayLength=1  InitialCondition=0
  Delay1 : Delay  DelayLength=1  InitialCondition=0
  Delay2 : Delay  DelayLength=1  InitialCondition=0
  Detect Fall Nonpositive : hdlsllib/Logic and Bit Operations/Detect Fall Nonpositive  vinit=0  OutDataTypeStr=boolean
  Detect Rise Positive : hdlsllib/Logic and Bit Operations/Detect Rise Positive  vinit=0  OutDataTypeStr=boolean
  Sample Control Bus Creator : whdlutilities/Sample Control Bus Creator
  data_out : Outport
  ctrl_out : Outport  Port=2
  wires:
  Detect Rise Positive/1 -> Sample Control Bus Creator/1
  Delay2/1 -> data_out/1
  data_in/1 -> Delay2/1
  Delay1/1 -> Detect Rise Positive/1
  Delay/1 -> Sample Control Bus Creator/3
  Sample Control Bus Creator/1 -> ctrl_out/1
  valid_in/1 -> Delay1/1, Detect Fall Nonpositive/1, Delay/1
  Detect Fall Nonpositive/1 -> Sample Control Bus Creator/2

== system rx2/process divide/transport_block1/Subsystem13/ctrl_gen ==
  data_in : Inport
  valid_in : Inport  Port=2
  Delay : Delay  DelayLength=1  InitialCondition=0
  Delay1 : Delay  DelayLength=1  InitialCondition=0
  Delay2 : Delay  DelayLength=1  InitialCondition=0
  Detect Fall Nonpositive : hdlsllib/Logic and Bit Operations/Detect Fall Nonpositive  vinit=0  OutDataTypeStr=boolean
  Detect Rise Positive : hdlsllib/Logic and Bit Operations/Detect Rise Positive  vinit=0  OutDataTypeStr=boolean
  Sample Control Bus Creator : whdlutilities/Sample Control Bus Creator
  data_out : Outport
  ctrl_out : Outport  Port=2
  wires:
  Detect Rise Positive/1 -> Sample Control Bus Creator/1
  Delay2/1 -> data_out/1
  data_in/1 -> Delay2/1
  Delay1/1 -> Detect Rise Positive/1
  Delay/1 -> Sample Control Bus Creator/3
  Sample Control Bus Creator/1 -> ctrl_out/1
  valid_in/1 -> Delay1/1, Detect Fall Nonpositive/1, Delay/1
  Detect Fall Nonpositive/1 -> Sample Control Bus Creator/2

== system rx2/process divide/transport_block1/Subsystem14/ctrl_gen ==
  data_in : Inport
  valid_in : Inport  Port=2
  Delay : Delay  DelayLength=1  InitialCondition=0
  Delay1 : Delay  DelayLength=1  InitialCondition=0
  Delay2 : Delay  DelayLength=1  InitialCondition=0
  Detect Fall Nonpositive : hdlsllib/Logic and Bit Operations/Detect Fall Nonpositive  vinit=0  OutDataTypeStr=boolean
  Detect Rise Positive : hdlsllib/Logic and Bit Operations/Detect Rise Positive  vinit=0  OutDataTypeStr=boolean
  Sample Control Bus Creator : whdlutilities/Sample Control Bus Creator
  data_out : Outport
  ctrl_out : Outport  Port=2
  wires:
  Detect Rise Positive/1 -> Sample Control Bus Creator/1
  Delay2/1 -> data_out/1
  data_in/1 -> Delay2/1
  Delay1/1 -> Detect Rise Positive/1
  Delay/1 -> Sample Control Bus Creator/3
  Sample Control Bus Creator/1 -> ctrl_out/1
  valid_in/1 -> Delay1/1, Detect Fall Nonpositive/1, Delay/1
  Detect Fall Nonpositive/1 -> Sample Control Bus Creator/2
